simulink model "Signaling_Model_Run"  (R2020b)
settings: configuration reference "VLS_Standard_RH850_Signalling" (kept outside this file)
libraries: simulink x1
settings Model: DataDictionary=Signaling_Sldd_test.sldd  Creator=mtarek-a  LastModifiedBy=amohsen2
settings ConfigSetRef: SourceName=VLS_Standard_RH850_Signalling

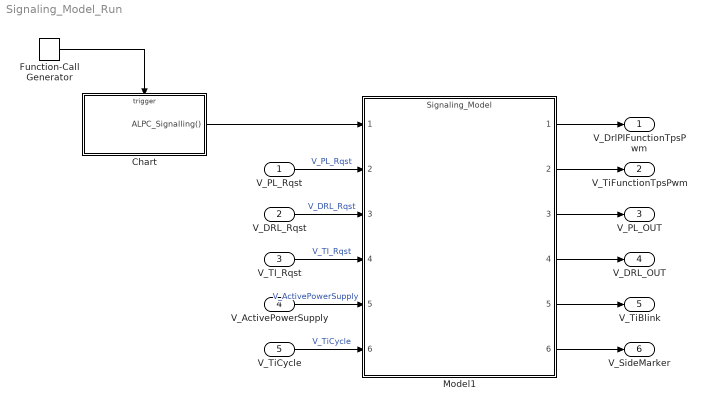
== system Signaling_Model_Run ==
  V_PL_Rqst : Inport
  V_DRL_Rqst : Inport  Port=2
  V_TI_Rqst : Inport  Port=3
  V_ActivePowerSupply : Inport  Port=4
  V_TiCycle : Inport  Port=5
  Chart : Stateflow chart  TreatAsAtomicUnit=on
  Function-Call Generator : simulink/Ports & Subsystems/Function-Call Generator  sample_time=0.02  numberOfIterations=1  DisallowWideOutput=off
  Model1 : ModelReference  ModelNameDialog=Signaling_Model.slx  SimulationMode=Normal  ScheduleRates=on  ModelReferenceVersion=1.149
  V_DrlPlFunctionTpsPwm : Outport
  V_TiFunctionTpsPwm : Outport  Port=2
  V_PL_OUT : Outport  Port=3
  V_DRL_OUT : Outport  Port=4
  V_TiBlink : Outport  Port=5
  V_SideMarker : Outport  Port=6
  wires:
  V_PL_Rqst/1 -> Model1/2  "V_PL_Rqst"
  Chart/1(ALPC_Signalling()) -> Model1/1
  V_DRL_Rqst/1 -> Model1/3  "V_DRL_Rqst"
  V_TI_Rqst/1 -> Model1/4  "V_TI_Rqst"
  V_ActivePowerSupply/1 -> Model1/5  "V_ActivePowerSupply"
  Function-Call Generator/1 -> Chart/Trigger
  V_TiCycle/1 -> Model1/6  "V_TiCycle"
  Model1/1 -> V_DrlPlFunctionTpsPwm/1
  Model1/2 -> V_TiFunctionTpsPwm/1
  Model1/3 -> V_PL_OUT/1
  Model1/4 -> V_DRL_OUT/1
  Model1/6 -> V_SideMarker/1
  Model1/5 -> V_TiBlink/1

== stateflow chart Signaling_Model_Run/Chart ==
  settings: executeAtInitialization=1
  state Scheduler
    on every(1,tik):
    send(ALPC_Signalling);
  (default) -> Scheduler
  events: ALPC_Signalling output FUNCTION_CALL_EVENT; tik input FUNCTION_CALL_EVENT
